simulink model "GlazedSolarCollector_ISO9806"  (R2018b)
settings: Solver=ode45  StartTime=0  StopTime=24*3600  MaxStep=600  RelTol=1e-3  EnableMultiTasking=on
InitFcn:
  | load('DE_TRY2010_13_averageYear')
undefined symbols (not defined in the file): path_carnot
libraries: carnot x15
settings Model: Creator=drhf  LastModifiedBy=drhf
settings DataIOCC: SaveFormat=Array  SignalLoggingSaveFormat=ModelDataLogs
settings OptimizationCC: ExpressionDepthLimit=2147483647  LifeSpan=inf
settings DebuggingCC: UnderspecifiedInitializationDetection=Classic  MergeDetectMultiDrivingBlocksExec=none  SolverPrmCheckMsg=warning  FcnCallInpInsideContextMsg=warning  StateNameClashWarn=warning  SFUnexpectedBacktrackingDiag=warning  SFNoUnconditionalDefaultTransitionDiag=warning  SFExecutionAtInitializationDiag=none
settings HardwareCC: ProdBitPerPointer=32  ProdBitPerSizeT=32  ProdBitPerPtrDiffT=32  ProdLargestAtomicFloat=None  ProdIntDivRoundTo=Undefined  ProdEndianess=Unspecified  ProdWordSize=32  ProdHWDeviceType=32-bit Generic
settings ModelReferenceCC: PropagateSignalLabelsOutOfModel=off
settings SFSimCC: SimUseLocalCustomCode=off
settings RTWCC: RTWUseLocalCustomCode=off
settings CodeAppCC: StateflowObjectComments=on
settings GRTTargetCC: TargetLangStandard=C89/C90 (ANSI)  GeneratePreprocessorConditionals=Disable all  CombineOutputUpdateFcns=off  GRTInterface=on
settings ConfigComp: CovMetricSettings=dw  CovHtmlReporting=on  CovSaveCumulativeToWorkspaceVar=on  CovSaveSingleToWorkspaceVar=on  CovExternalEMLEnable=off

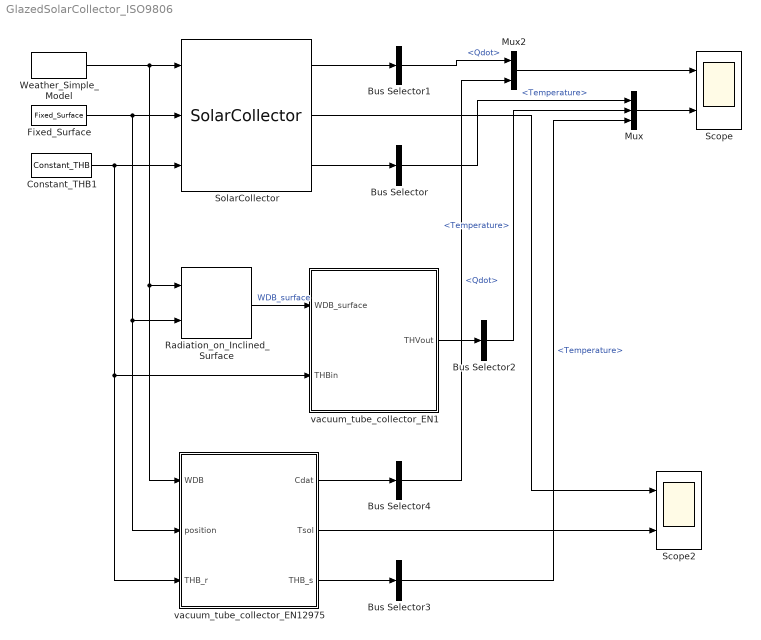
== system GlazedSolarCollector_ISO9806 ==
  Bus Selector : BusSelector  OutputSignals=Temperature
  Bus Selector1 : BusSelector  OutputSignals=Qdot
  Bus Selector2 : BusSelector  OutputSignals=Temperature
  Bus Selector3 : BusSelector  OutputSignals=Temperature
  Bus Selector4 : BusSelector  OutputSignals=Qdot
  Constant_THB1 : carnot/Source/Simple/Constant_THB  t=40  mdot=100/3600  p=1e5  mID=Full Pressure Drop with Static Height  fluid=Water  mix=0  mix2=0  mix3=0  dia=0.02  hgt=0
      settings: SourceProductName=Carnot
  Fixed_Surface : carnot/Weather/Fixed_Surface  colangle=30  colazi=0  colrot=0
      settings: SourceProductName=Carnot
  Mux : Mux  Inputs=3
  Mux2 : Mux  Inputs=2
  Radiation_on_Inclined_Surface : carnot/Weather/Radiation_on_Inclined_Surface  sky=Perez 1990  reflect=0.2
      settings: SourceProductName=Carnot
  Scope : Scope  NumInputPorts=2
  Scope2 : Scope  NumInputPorts=2
  SolarCollector : carnot/Source/Solar_Thermal/SolarCollector  t0=20  Ncollector=2  PathName=fullfile(path_carnot('libsl'), 'Source', 'Solar_Thermal', 'SolarCollector', 'parameter_set')  FileName='DefaultCollector.mat'  userPath=off  userParam=off  acol=3.5  len=0.1  fta=0.7  c1=1.1  c2=0.001  c3=0  c4=0  c5=5000  c6=0  KbAngles=[0 5 10 15 20 25 30 35 40 45 50 55 60 65 70 75 80 85 90]  KbL=[1 1 0.9999 0.9996 0.9991 0.9982 0.9965 0.9935 0.9886 0.9807 0.9678 0.9473 0.9148 0.8638 0.7846 0.6644 0.4907 0.2599 0]  KbT=[1 1 1 1 1 1 1 1 1 1 1 0.875 0.75 0.625 0.5 0.375 0.25 0.125 0]  Kd=0.92  dplin=10  dpqua=10  SensorTimeConstant=10
      settings: SourceProductName=Carnot
  Weather_Simple_Model : carnot/Weather/Weather_Simple_Model  Ibn=900  Idg=100  tamb=5  deltaTsky=-6  rh=50  precip="10e-3/24/3600           % 10 mm in 24 h"  cloud=0.125  p=1013e2  vw=1  wdir=270  lat=60  colangle=0  colazi=0  colrot=0
      settings: SourceProductName=Carnot
  vacuum_tube_collector_EN1 : Subsystem  mask(collector){acol=7, c1=1.1, c2=0.001, c3=0, c4=0, c5=5000, c6=0, fta=0.7, kblangle=[0 5 10 15 20 25 30 35 40 45 50 55 60 65 70 75 80 85 90], KbL=[1 1 0.9999 0.9996 0.9991 0.9982 0.9965 0.9935 0.9886 0.9807 0.9678 0.9473 0.9148 0.8638 0.7846 0.6644 0.4907 0.2599 0], KbT=[1 1 1 1 1 1 1 1 1 1 1 0.875 0.75 0.625 0.5 0.375 0.25 0.125 0], Kd=0.92, len=0.1, tini=20}
      mask prompts: acol "A : collector surface  [m²]"; c1 "c1 : heat loss coefficient at (Tm-Ta)=0  [W/(m²*K)]"; c2 "c2: temperature dependence of the heat loss coefficient [W/(m*K)²]"; c3 "c3 : wind speed dependence of the heat loss coefficient [J/(m³K)]"; c4 "c4 : sky temperature dependence of the heat loss coefficient [W/(m²K)]"; c5 "c5 : effective thermal capacity [J/(m²K)]"; c6 "c6 : wind dependence in the zero loss efficiency [s/m]"; fta "Fin Efficiency * Transmission * Absorption (F'(tau alfa))"; kblangle "KbL: angles for longitudinal IAM [degree]"; KbL "KbL: values for longitudinal incidence angle modifier (0..1)"; KbT "KbT: values for transversal incidence angle modifier (0..1)"; Kd "Kd : Incidence angle modifier diffuse radiation"; len "length between inlet and outlet [m]"; tini "initial temperature [degree centigrade]"
      mask help:
      | Collector model according to EN 12975 standard.
      | Energy balance:
      | mdot cp (Tout-Tin) /A = F'(TauAlfa) Kdir Idir + F'(TauAlfa) Kdfu Idfu
      |        - c1 (Tm-Tamb) - c2 (Tm-Tamb)^2 - c3 v_wind (Tm-Ta) - c6 v_wind Iglb
      |        + c4 (ELongwave - sigmaSB*(Tamb+273.15)^4) - c5 dTm/dt
      |
      | Often in test reports the optical efficiency or conversion factor eta0 is given.
      | The correlation for F'(TauAlfa) is:
      | eta0 = F'(TauAlfa) * (Kdir(15°)*0.85 + Kdfu*0.15)
      | or
      | F'(TauAlfa) = eta0 / (Kdir(15°)*0.85 + Kdfu*0.15)
      mask init:
      | acol = max(acol, 0.01);
      | c5 = max(c5, 0.001);
      mask Help: eval('htmlhelp (''chap_4_2c.htm#collector_flat_plate'')')
      mask TypeOptions fta: IAM_Table_KbL_KbT/fta
      mask TypeOptions kblangle: IAM_Table_KbL_KbT/kblangle | IAM_Table_KbL_KbT/kbtangle
      mask TypeOptions KbL: IAM_Table_KbL_KbT/KbL
      mask TypeOptions KbT: IAM_Table_KbL_KbT/KbT
      mask TypeOptions Kd: IAM_Table_KbL_KbT/Kd
      mask Display: disp('solar thermal\nflat plate\ncollector\nEN 12975')
  vacuum_tube_collector_EN12975 : Subsystem  mask(Solar Thermal Collector){t0=20, Ncollector=2, PathName=fullfile(path_carnot('libsl'), 'Source', 'Solar_Thermal', 'SolarCollector', 'parameter_set'), FileName='DefaultCollector.mat', userPath=off, userParam=off, acol=3.5, len=0.1, fta=0.7, c1=1.1, c2=0.001, c3=0, c4=0, c5=5000, c6=0, KbAngles=[0 5 10 15 20 25 30 35 40 45 50 55 60 65 70 75 80 85 90], KbL=[1 1 0.9999 0.9996 0.9991 0.9982 0.9965 0.9935 0.9886 0.9807 0.9678 0.9473 0.9148 0.8638 0.7846 0.6644 0.4907 0.2599 0], KbT=[1 1 1 1 1 1 1 1 1 1 1 0.875 0.75 0.625 0.5 0.375 0.25 0.125 0], Kd=0.92, dplin=10, dpqua=10, SensorTimeConstant=10}
      mask prompts: t0 "Initial temperature [°C]"; Ncollector "Number of collectors in parallel"; PathName "Path"; FileName "Parameter set"; userPath "Edit path and name of parameter set"; userParam "User defined parameters"; acol "A: surface  of one collector module in m²"; len "Length between collector inlet and outlet in m"; fta "Fin Efficiency * Transmission * Absorption (F'(tau alfa))"; c1 "c1 : heat loss coefficient at (Tm-Ta)=0  [W/(m²*K)]"; c2 "c2: temperature dependence of the heat loss coefficient [W/(m*K)²]"; c3 "c3 : wind speed dependence of the heat loss coefficient [J/(m³K)]"; c4 "c4 : sky temperature dependence of the heat loss coefficient [W/(m²K)]"; c5 "c5 : effective thermal capacity [J/(m²K)]"; c6 "c6 : wind dependence in the zero loss efficiency [s/m]"; KbAngles "Kb: angles for longitudinal and transversal IAM [degree]"; KbL "KbL: values for longitudinal incidence angle modifier (0..1)"; KbT "KbT: values for transversal incidence angle modifier (0..1)"; Kd "Kd : Incidence angle modifier diffuse radiation"; dplin "lin: linear pressure drop in Pa/(kg/s)"; dpqua "qua: quadratic pressure drop in Pa/(kg/s)²"; SensorTimeConstant "time constant of sensor [s]"
      mask help: Dynamic 1-node solar thermal collector model according to ISO 9806 standard. Collector optics use a lookup table for the incidence angle modifier. Especially tube collectors have asymmetric IAM and require a geometry dependancy.
      mask init:
      | % callback to set parameters of model
      | [ok, param] = CarnotCallbacks_CollectorEN12975Conf('SetParameters',gcbh,PathName,FileName);
      mask Help: web(fullfile(path_carnot('help'),'collector_en12975.html'),'-helpbrowser')
      mask TypeOptions t0: T_Sensor/t0 | solar_collector_basic/tini
      mask TypeOptions Ncollector: Ncollector/Value | Gain1/Gain | Gain2/Gain
      mask Callback userPath: [ok, param] = CarnotCallbacks_CollectorEN12975Conf('UserEdit',gcbh);
      mask Callback userParam: [ok, param] = CarnotCallbacks_CollectorEN12975Conf('UserEdit',gcbh);
      mask TypeOptions acol: solar_collector_basic/acol | Acol/Value
      mask TypeOptions len: Pressure_Drop_Collector/len
      mask TypeOptions fta: IAM_Table_KbL_KbT/fta
      mask TypeOptions c1: solar_collector_basic/c1
      mask TypeOptions c2: solar_collector_basic/c2
      mask TypeOptions c3: solar_collector_basic/c3
      mask TypeOptions c4: solar_collector_basic/c4
      mask TypeOptions c5: solar_collector_basic/c5
      mask TypeOptions c6: solar_collector_basic/c6
      mask TypeOptions KbAngles: IAM_Table_KbL_KbT/kblangle | IAM_Table_KbL_KbT/kbtangle
      mask TypeOptions KbL: IAM_Table_KbL_KbT/KbL
      mask TypeOptions KbT: IAM_Table_KbL_KbT/KbT
      mask TypeOptions Kd: IAM_Table_KbL_KbT/Kd
      mask TypeOptions dplin: Pressure_Drop_Collector/lin
      mask TypeOptions dpqua: Pressure_Drop_Collector/qua
      mask TypeOptions SensorTimeConstant: T_Sensor/tc
      mask DialogControl ParameterGroupVar Prompt: Picking a parameter set
      mask DialogControl Control2 Prompt: Carnot public data
      mask DialogControl Control2 Callback: [ok, file] = CarnotCallbacks_CollectorEN12975Conf('GetFilename',gcbh,'public');
      mask DialogControl Control3 Prompt: Carnot internal data
      mask DialogControl Control3 Callback: [ok, file] = CarnotCallbacks_CollectorEN12975Conf('GetFilename',gcbh,'internal');
      mask DialogControl Control4 Prompt: Selected path
      mask DialogControl Control4 Callback: [ok, file] = CarnotCallbacks_CollectorEN12975Conf('GetFilename',gcbh,'selected');
      mask DialogControl Container7 Prompt: Geometry
      mask DialogControl Container8 Prompt: Coll.Params
      mask DialogControl Container9 Prompt: Optics
      mask DialogControl Container10 Prompt: Hydraulic
      mask DialogControl Container11 Prompt: Sensors
      mask DialogControl Control5 Prompt: Save in Carnot interal data
      mask DialogControl Control5 Callback: [ok, param] = CarnotCallbacks_CollectorEN12975Conf('SaveFilename',gcbh,'internal','COL');
      mask DialogControl Control6 Prompt: Save in seleced path
      mask DialogControl Control6 Callback: [ok, param] = CarnotCallbacks_CollectorEN12975Conf('SaveFilename',gcbh,'selected','COL');
      mask Display:
      | % user defined picture file
      | picfile = fullfile(path_carnot('intlibsl'), ...
      |     'Source','Solar_Thermal','SolarCollector','parameter_set', ...
      |      'Collector_CONF.jpg');
      | 
      | pic = false;
      | 
      | % show internal picture if defined
      | if ~BlockIsInCarnotLibrary    % if not located in library any more
      |     if exist(picfile)
      |         image(imread(picfile), [0.2, 0, 0.6, 1])
      |         set_param(gcb, 'BackgroundColor', 'White')
      |         pic = true;
      |     end
      | end
      | 
      | if ~pic    % show public picture
      |     disp('Solar Thermal\nCollector\n\nISO 9806')
      |     set_param(gcb, 'BackgroundColor', 'Yellow')
      | end
  wires:
  Weather_Simple_Model/1 -> SolarCollector/1, vacuum_tube_collector_EN12975/1(WDB), Radiation_on_Inclined_Surface/1
  Constant_THB1/1 -> SolarCollector/3, vacuum_tube_collector_EN12975/3(THB_r), vacuum_tube_collector_EN1/2(THBin)
  Fixed_Surface/1 -> SolarCollector/2, vacuum_tube_collector_EN12975/2(position), Radiation_on_Inclined_Surface/2
  SolarCollector/1 -> Bus Selector1/1
  Bus Selector/1 -> Mux/1  "<Temperature>"
  Bus Selector1/1 -> Mux2/1  "<Qdot>"
  SolarCollector/3 -> Bus Selector/1
  SolarCollector/2 -> Scope2/1
  Mux/1 -> Scope/2
  Radiation_on_Inclined_Surface/1 -> vacuum_tube_collector_EN1/1(WDB_surface)  "WDB_surface"
  vacuum_tube_collector_EN1/1(THVout) -> Bus Selector2/1
  Bus Selector2/1 -> Mux/2  "<Temperature>"
  vacuum_tube_collector_EN12975/3(THB_s) -> Bus Selector3/1
  Bus Selector3/1 -> Mux/3  "<Temperature>"
  vacuum_tube_collector_EN12975/1(Cdat) -> Bus Selector4/1
  vacuum_tube_collector_EN12975/2(Tsol) -> Scope2/2
  Bus Selector4/1 -> Mux2/2  "<Qdot>"
  Mux2/1 -> Scope/1

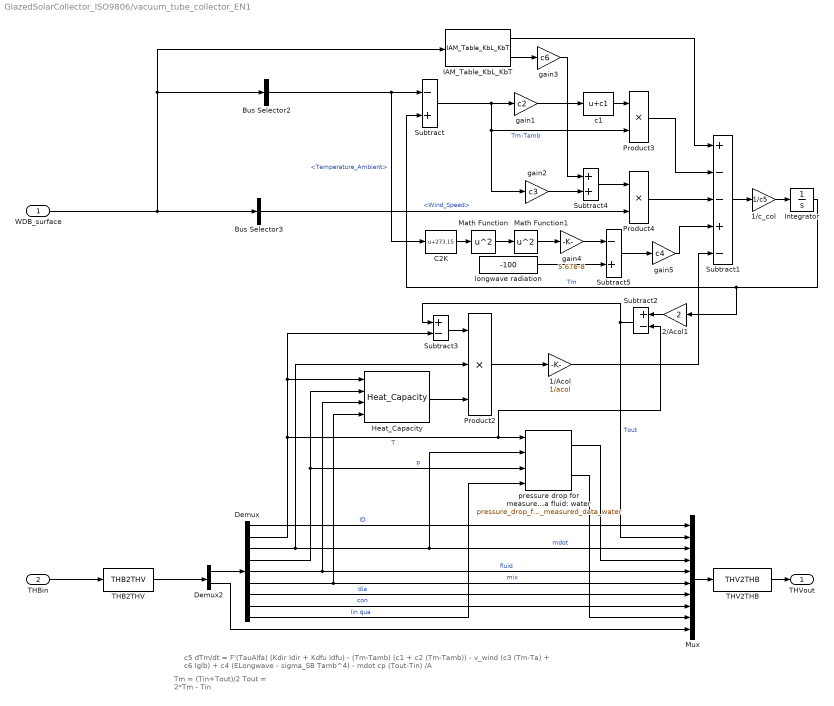
== system GlazedSolarCollector_ISO9806/vacuum_tube_collector_EN1 ==
  note: c5 dTm/dt = F'(TauAlfa) (Kdir Idir + Kdfu Idfu) - (Tm-Tamb) (c1 + c2 (Tm-Tamb)) - v_wind (c3 (Tm-Ta) + c6 Iglb) + c4 (ELongwave - sigma_SB Tamb^4) - mdot cp (Tout-Tin) /A
  note: Tm = (Tin+Tout)/2
      | Tout = 2*Tm - Tin
  WDB_surface : Inport
  THBin : Inport  Port=2
  1/Acol : Gain  Gain=1/acol
  1/c_col : Gain  Gain=1/c5
  2/Acol1 : Gain  Gain=2
  Bus Selector2 : BusSelector  OutputSignals=Temperature_Ambient
  Bus Selector3 : BusSelector  OutputSignals=Wind_Speed
  C2K : Bias  Bias=273.15
  Demux : Demux  Outputs=[1 1 1 1 1 1 1 1 2]
  Demux2 : Demux  Outputs=[10 -1]
  Heat_Capacity : carnot/Basic/Material_Properties/Heat_Capacity  VariantControl=CarlibClassic  INPUTARGUMENTS=state variables (classic)  DEBUGLEVEL=DEBUGLEVEL  MAXTOTALWARNINGS=inf  MAXCONSECUTIVEWARNINGS=inf  WRITETOFILE=0  FILENAME='errors.txt'
      settings: SourceProductName=Carnot
  IAM_Table_KbL_KbT : carnot/Source/Solar_Thermal/IncidenceAngleModifier/IAM_Table_KbL_KbT  fta=fta  kblangle=kblangle  KbL=KbL  kbtangle=kblangle  KbT=KbT  Kd=Kd
      settings: SourceProductName=Carnot
  Integrator : Integrator  InitialCondition=tini
  Math Function : Math  Operator=square  SaturateOnIntegerOverflow=on
  Math Function1 : Math  Operator=square  SaturateOnIntegerOverflow=on
  Mux : Mux  Inputs=10
  Product2 : Product  Inputs=3  RndMeth=Zero
  Product3 : Product  RndMeth=Zero
  Product4 : Product  RndMeth=Zero
  Subtract : Sum  Inputs=-+
  Subtract1 : Sum  Inputs=+--+-
  Subtract2 : Sum  Inputs=+-
  Subtract3 : Sum  Inputs=+-
  Subtract4 : Sum  Inputs=2
  Subtract5 : Sum  Inputs=-+
  THB2THV : carnot/Toolbox/THB2THV
      settings: SourceProductName=Carnot
  THV2THB : carnot/Toolbox/THV2THB
      settings: SourceProductName=Carnot
  c1 : Bias  Bias=c1
  gain1 : Gain  Gain=c2
  gain2 : Gain  Gain=c3
  gain3 : Gain  Gain=c6
  gain4 : Gain  Gain=5.67e-8
  gain5 : Gain  Gain=c4
  longwave radiation : Constant  Value=-100
  pressure drop for measured data fluid: water : carnot/Source/Solar_Thermal/PressureDropCollector/pressure_drop_for_measured_data_water  mdottest=0.01*1.96  ttest=20  pdroptest=158*1.96  aonecol=1.96  acol=acol
      settings: SourceProductName=Carnot
  THVout : Outport  InitialOutput=0
  wires:
  Demux/3 -> pressure drop for measured data fluid: water/2, Mux/3, Product2/2  "mdot"
  Demux/5 -> Heat_Capacity/3, Mux/5  "fluid"
  Demux/1 -> Mux/1  "ID"
  Demux2/1 -> Demux/1
  THBin/1 -> THB2THV/1
  Demux/4 -> pressure drop for measured data fluid: water/3, Heat_Capacity/2  "p"
  Demux/6 -> Heat_Capacity/4, Mux/6  "mix"
  pressure drop for measured data fluid: water/1 -> Mux/4
  pressure drop for measured data fluid: water/2 -> Mux/9
  Demux/9 -> pressure drop for measured data fluid: water/4  "lin qua"
  Demux/8 -> Mux/8  "con"
  Demux/7 -> Mux/7  "dia"
  Demux2/2 -> Mux/10
  Demux/2 -> Heat_Capacity/1, Subtract3/2, pressure drop for measured data fluid: water/1, Subtract2/2  "T"
  Bus Selector2/1 -> C2K/1, Subtract/1  "<Temperature_Ambient>"
  Subtract1/1 -> 1/c_col/1
  1/c_col/1 -> Integrator/1
  Heat_Capacity/1 -> Product2/3
  Product2/1 -> 1/Acol/1
  Integrator/1 -> 2/Acol1/1, Subtract/2  "Tm"
  Subtract3/1 -> Product2/1
  Subtract/1 -> gain1/1, Product3/2, gain2/1  "Tm-Tamb"
  IAM_Table_KbL_KbT/1 -> Subtract1/1
  gain1/1 -> c1/1
  c1/1 -> Product3/1
  Product3/1 -> Subtract1/2
  gain2/1 -> Subtract4/2
  IAM_Table_KbL_KbT/2 -> gain3/1
  gain3/1 -> Subtract4/1
  Product4/1 -> Subtract1/3
  Subtract4/1 -> Product4/1
  Bus Selector3/1 -> Product4/2  "<Wind_Speed>"
  Math Function/1 -> Math Function1/1
  C2K/1 -> Math Function/1
  Math Function1/1 -> gain4/1
  gain4/1 -> Subtract5/1
  longwave radiation/1 -> Subtract5/2
  1/Acol/1 -> Subtract1/5
  Subtract5/1 -> gain5/1
  gain5/1 -> Subtract1/4
  Subtract2/1 -> Mux/2, Subtract3/1  "Tout"
  2/Acol1/1 -> Subtract2/1
  THB2THV/1 -> Demux2/1
  THV2THB/1 -> THVout/1
  Mux/1 -> THV2THB/1
  WDB_surface/1 -> Bus Selector3/1, IAM_Table_KbL_KbT/1, Bus Selector2/1

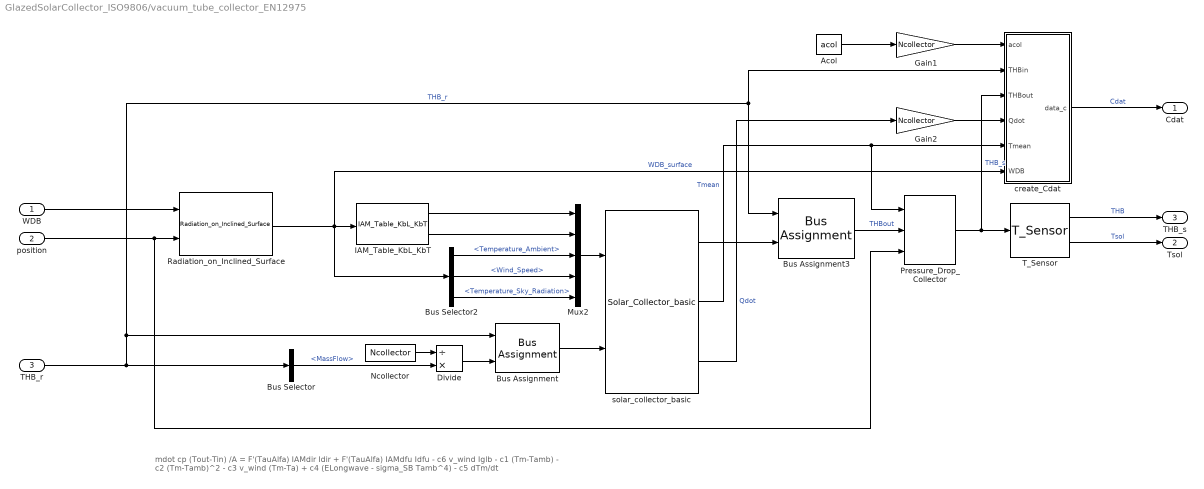
== system GlazedSolarCollector_ISO9806/vacuum_tube_collector_EN12975 ==
  note: mdot cp (Tout-Tin) /A = F'(TauAlfa) IAMdir Idir + F'(TauAlfa) IAMdfu Idfu - c6 v_wind Iglb - c1 (Tm-Tamb) - c2 (Tm-Tamb)^2 - c3 v_wind (Tm-Ta) + c4 (ELongwave - sigma_SB Tamb^4) - c5 dTm/dt
  WDB : Inport
  position : Inport  Port=2
  THB_r : Inport  Port=3
  Acol : Constant  Value=acol
  Bus Assignment : BusAssignment  AssignedSignals=MassFlow
  Bus Assignment3 : BusAssignment  AssignedSignals=Temperature
  Bus Selector : BusSelector  OutputSignals=MassFlow
  Bus Selector2 : BusSelector  OutputSignals=Temperature_Ambient,Wind_Speed,Temperature_Sky_Radiation
  Divide : Product  Inputs=/*
  Gain1 : Gain  Gain=Ncollector
  Gain2 : Gain  Gain=Ncollector
  IAM_Table_KbL_KbT : carnot/Source/Solar_Thermal/IncidenceAngleModifier/IAM_Table_KbL_KbT  fta=fta  kblangle=KbAngles  KbL=KbL  kbtangle=KbAngles  KbT=KbT  Kd=Kd
      settings: SourceProductName=Carnot
  Mux2 : Mux  Inputs=5
  Ncollector : Constant  Value=Ncollector
  Pressure_Drop_Collector : carnot/Basic/Pressure_Drop/Pressure_Drop_Collector  len=len  lin=dplin  qua=dpqua
      settings: SourceProductName=Carnot
  Radiation_on_Inclined_Surface : carnot/Weather/Radiation_on_Inclined_Surface  sky=Perez 1990  reflect=0.2
      settings: SourceProductName=Carnot
  T_Sensor : carnot/Control/T_Sensor  tc=SensorTimeConstant  t0=t0
      settings: SourceProductName=Carnot
  create_Cdat : Subsystem
  solar_collector_basic : carnot/Basic/Thermal_Models/Solar_Collector_basic  acol=acol  c1=c1  c2=c2  c3=c3  c4=c4  c5=c5  c6=c6  tini=t0
      settings: SourceProductName=Carnot
  Cdat : Outport
  Tsol : Outport  Port=2
  THB_s : Outport  Port=3
  wires:
  T_Sensor/1 -> THB_s/1  "THB"
  T_Sensor/2 -> Tsol/1  "Tsol"
  Divide/1 -> Bus Assignment/2
  Ncollector/1 -> Divide/1
  Bus Assignment/1 -> solar_collector_basic/2
  WDB/1 -> Radiation_on_Inclined_Surface/1
  solar_collector_basic/3 -> Gain2/1  "Qdot"
  Bus Assignment3/1 -> Pressure_Drop_Collector/2  "THBout"
  THB_r/1 -> Bus Selector/1, create_Cdat/2(THBin), Bus Assignment3/1, Bus Assignment/1  "THB_r"
  solar_collector_basic/1 -> Bus Assignment3/2
  solar_collector_basic/2 -> create_Cdat/5(Tmean), Pressure_Drop_Collector/1  "Tmean"
  IAM_Table_KbL_KbT/2 -> Mux2/2
  Bus Selector2/3 -> Mux2/5  "<Temperature_Sky_Radiation>"
  create_Cdat/1(data_c) -> Cdat/1  "Cdat"
  Radiation_on_Inclined_Surface/1 -> create_Cdat/6(WDB), Bus Selector2/1, IAM_Table_KbL_KbT/1  "WDB_surface"
  Mux2/1 -> solar_collector_basic/1
  Bus Selector2/1 -> Mux2/3  "<Temperature_Ambient>"
  Pressure_Drop_Collector/1 -> create_Cdat/3(THBout), T_Sensor/1  "THB_s"
  IAM_Table_KbL_KbT/1 -> Mux2/1
  Bus Selector2/2 -> Mux2/4  "<Wind_Speed>"
  position/1 -> Pressure_Drop_Collector/3, Radiation_on_Inclined_Surface/2
  Acol/1 -> Gain1/1
  Bus Selector/1 -> Divide/2  "<MassFlow>"
  Gain1/1 -> create_Cdat/1(acol)
  Gain2/1 -> create_Cdat/4(Qdot)

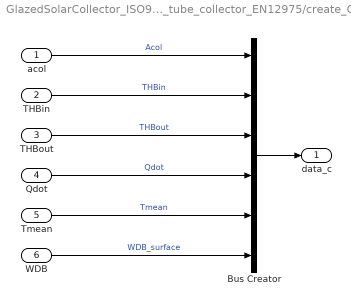
== system GlazedSolarCollector_ISO9806/vacuum_tube_collector_EN12975/create_Cdat ==
  acol : Inport
  THBin : Inport  Port=2
  THBout : Inport  Port=3
  Qdot : Inport  Port=4
  Tmean : Inport  Port=5
  WDB : Inport  Port=6
  Bus Creator : BusCreator  Inputs=6
  data_c : Outport
  wires:
  Tmean/1 -> Bus Creator/5  "Tmean"
  Qdot/1 -> Bus Creator/4  "Qdot"
  Bus Creator/1 -> data_c/1
  WDB/1 -> Bus Creator/6  "WDB_surface"
  THBout/1 -> Bus Creator/3  "THBout"
  THBin/1 -> Bus Creator/2  "THBin"
  acol/1 -> Bus Creator/1  "Acol"
